simulink library "mbdriLib"  (R2021b)
settings: Solver=ode45  StartTime=0.0  StopTime=10.0  RelTol=1e-3  EnableMultiTasking=on
undefined symbols (not defined in the file or in its folder): ap, deg, DiscIntNeverNeededParam, Earth, env, flat2lla, Newton, rad, Raphson, s, uavData, WGS84, Xpoints, Ypoints, Zpoints
libraries: simulink x23, $bdroot x7, aerolibconvert2 x2, slpidlib x1, sharedtransform x1, SignalEditorBlockLib x1, aerolibtransform2 x1
(part 2 of 2)

== matlab function mbdriLib/Filtering/RateAid for GPS ==
  data: u input size=1; y output size=1; NewGPS input size=1; Ts input size=1 =Ts
function y = RateAid(u,NewGPS,Ts)
persistent LastU;
persistent TimeSinceLast;
persistent rate;
persistent OldRate;

if (isempty(LastU))
    LastU = 0;
    TimeSinceLast = Ts;
    rate = 0;
    OldRate = 0;
end

if (NewGPS)
    OldRate = rate;
    rate = (u - LastU)/TimeSinceLast;
    TimeSinceLast = 0;
    LastU = u;
end
y = u + ( .5*rate + .5*OldRate )*TimeSinceLast;
TimeSinceLast = TimeSinceLast + Ts;
